simulink library "libMultiPacket"  (R2013b)
settings: Solver=ode45  StartTime=0.0  StopTime=10.0  RelTol=1e-3
undefined symbols (not defined in the file): macaddr
libraries: xpcutilitieslib x2, simulink x1, dspindex x1, libNetwork x1, xpcethernetlib x1, libSerialize x1
settings Model: Creator=djoshea  LastModifiedBy=djoshea

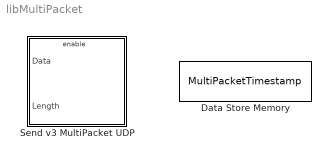
== system libMultiPacket ==
  Data Store Memory : DataStoreMemory  DataStoreName=MultiPacketTimestamp  ReadBeforeWriteMsg=warning  WriteAfterWriteMsg=warning  WriteAfterReadMsg=warning  OutDataTypeStr=double
  Send v3 MultiPacket UDP : Subsystem  mask{transmitId=1, sourceIP=[192 168 1 1], sourcePort=10000, destIP=[192 168 1 255], destPort=28000, DstMac=macaddr('ff:ff:ff:ff:ff:ff'), ID=1}
      mask prompts: transmitId "Transmit Block Id"; sourceIP "Source IP"; sourcePort "Source Port"; destIP "Dest IP"; destPort "Dest Port"; DstMac "Dest MAC"; ID "Ethernet Tx Id"
      mask TypeOptions sourceIP: Mask provides bytesPerPacket/sourceIP
      mask TypeOptions sourcePort: Mask provides bytesPerPacket/sourcePort
      mask TypeOptions destIP: Mask provides bytesPerPacket/destIP
      mask TypeOptions destPort: Mask provides bytesPerPacket/destPort
      mask TypeOptions DstMac: Mask provides bytesPerPacket/DstMac
      mask TypeOptions ID: Mask provides bytesPerPacket/ID

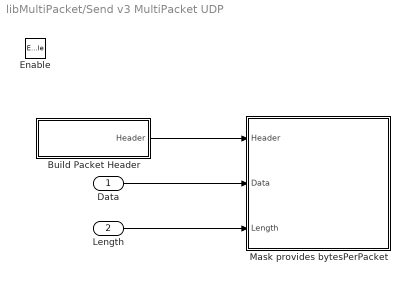
== system libMultiPacket/Send v3 MultiPacket UDP ==
  Data : Inport
  Length : Inport  Port=2  OutDataTypeStr=uint16
  Enable : EnablePort
  Build Packet Header : Subsystem
  Mask provides bytesPerPacket : Subsystem  mask{bytesPerPacket=1472-4-14, ID=1, sourceIP=sourceIP, sourcePort=10000, destIP=destIP, destPort=28000, DstMac=macaddr('ff:ff:ff:ff:ff:ff')}
      mask prompts: ID "Ethernet Tx Id"; sourceIP "Source IP"; sourcePort "Source Port"; destIP "Dest IP"; destPort "Dest Port"; DstMac "Dest MAC"
      mask TypeOptions ID: Packet Send Iterator/ID
      mask TypeOptions sourceIP: Packet Send Iterator/sourceIP
      mask TypeOptions sourcePort: Packet Send Iterator/sourcePort
      mask TypeOptions destIP: Packet Send Iterator/destIP
      mask TypeOptions destPort: Packet Send Iterator/destPort
      mask TypeOptions DstMac: Packet Send Iterator/DstMac
  wires:
  Build Packet Header/1(Header) -> Mask provides bytesPerPacket/1(Header)
  Length/1 -> Mask provides bytesPerPacket/3(Length)
  Data/1 -> Mask provides bytesPerPacket/2(Data)

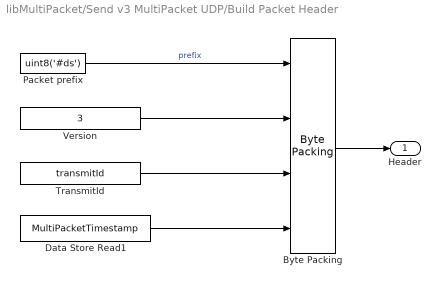
== system libMultiPacket/Send v3 MultiPacket UDP/Build Packet Header ==
  "Byte Packing " : xpcutilitieslib/Byte Packing   MaskPackedDataType=uint8  MaskUnpackedDataTypes={'uint8','uint16', 'uint8', 'double'}  MaskAlignment=1
  Data Store Read1 : DataStoreRead  DataStoreName=MultiPacketTimestamp
  Packet prefix : Constant  Value=uint8('#ds')  OutDataTypeStr=uint8
  TransmitId : Constant  Value=transmitId  OutDataTypeStr=uint8
  Version : Constant  Value=3  OutDataTypeStr=uint16
  Header : Outport
  wires:
  "Byte Packing "/1 -> Header/1
  Packet prefix/1 -> "Byte Packing "/1  "prefix"
  Version/1 -> "Byte Packing "/2
  Data Store Read1/1 -> "Byte Packing "/4
  TransmitId/1 -> "Byte Packing "/3

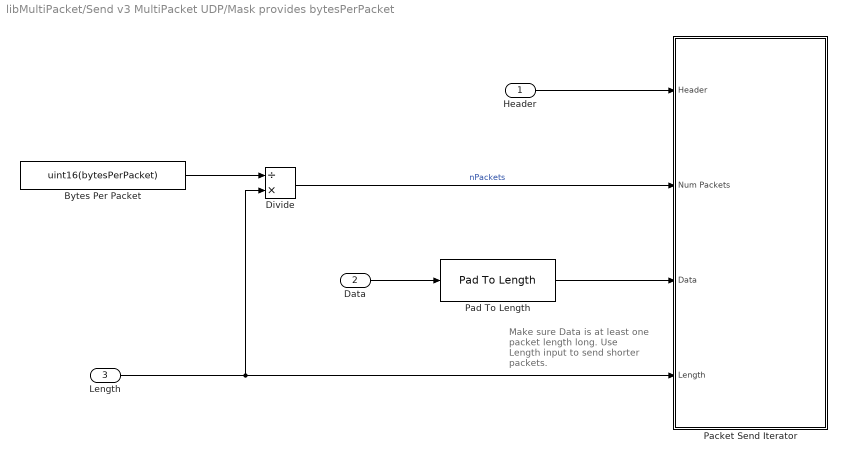
== system libMultiPacket/Send v3 MultiPacket UDP/Mask provides bytesPerPacket ==
  note: Make sure Data is at least one packet length long.
      | Use Length input to send shorter packets.
  Header : Inport
  Data : Inport  Port=2
  Length : Inport  Port=3  OutDataTypeStr=uint16
  Bytes Per Packet : Constant  Value=uint16(bytesPerPacket)  OutDataTypeStr=uint16
  Divide : Product  Inputs=/*  OutDataTypeStr=uint16  RndMeth=Ceiling
  Packet Send Iterator : Subsystem  TreatAsAtomicUnit=on  mask{bytesPerPacket=bytesPerPacket, ID=1, sourceIP=sourceIP, sourcePort=10000, destIP=destIP, destPort=28000, DstMac=macaddr('ff:ff:ff:ff:ff:ff')}
      mask prompts: bytesPerPacket "Bytes per Packet"; ID "Ethernet Tx Id"; sourceIP "Source IP"; sourcePort "Source Port"; destIP "Dest IP"; destPort "Dest Port"; DstMac "Dest MAC"
      mask TypeOptions ID: Send UDP/ID
      mask TypeOptions sourceIP: Send UDP/sourceIP
      mask TypeOptions sourcePort: Send UDP/sourcePort
      mask TypeOptions destIP: Send UDP/destIP
      mask TypeOptions destPort: Send UDP/destPort
      mask TypeOptions DstMac: Send UDP/DstMac
  Pad To Length : libSerialize/Pad To Length  bufferMinSize=bytesPerPacket
  wires:
  Header/1 -> Packet Send Iterator/1(Header)
  Pad To Length/1 -> Packet Send Iterator/3(Data)
  Divide/1 -> Packet Send Iterator/2(Num Packets)  "nPackets"
  Length/1 -> Packet Send Iterator/4(Length), Divide/2
  Bytes Per Packet/1 -> Divide/1
  Data/1 -> Pad To Length/1

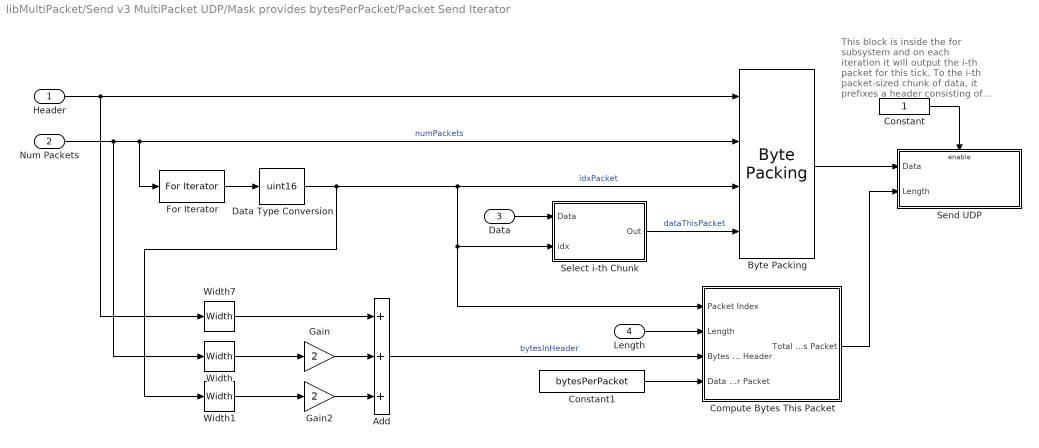
== system libMultiPacket/Send v3 MultiPacket UDP/Mask provides bytesPerPacket/Packet Send Iterator ==
  note: This block is inside the for subsystem and on each iteration
      | it will output the i-th packet for this tick. To the i-th packet-sized
      |  chunk of data, it prefixes a header consisting of a version, total
      |  packet count, and packet index.
  Header : Inport  OutDataTypeStr=uint8
  Num Packets : Inport  Port=2  OutDataTypeStr=uint16
  Data : Inport  Port=3  OutDataTypeStr=uint8
  Length : Inport  Port=4  OutDataTypeStr=uint16
  Add : Sum  Inputs=+++  OutDataTypeStr=uint16
  "Byte Packing " : xpcutilitieslib/Byte Packing   MaskPackedDataType=uint8  MaskUnpackedDataTypes={'uint8', 'uint16', 'uint16', 'uint8'}  MaskAlignment=1
  Compute Bytes This Packet : Subsystem
  Constant : Constant  OutDataTypeStr=Inherit: Inherit via back propagation
  Constant1 : Constant  Value=bytesPerPacket  OutDataTypeStr=uint16
  Data Type Conversion : DataTypeConversion  OutDataTypeStr=uint16
  For Iterator : ForIterator  IterationSource=external  IterationVariableDataType=int16
  Gain : Gain  Gain=2  OutDataTypeStr=uint16
  Gain2 : Gain  Gain=2  OutDataTypeStr=uint16
  Select i-th Chunk : Subsystem  mask{elementsPerChunk=bytesPerPacket}
      mask prompts: elementsPerChunk "Elements Per Chunk"
  Send UDP : Subsystem  mask{sourceIP=sourceIP, sourcePort=10000, destIP=destIP, destPort=28000, DstMac=macaddr('ff:ff:ff:ff:ff:ff'), ID=1}
      mask prompts: sourceIP "Source IP"; sourcePort "Source Port"; destIP "Dest IP"; destPort "Dest Port"; DstMac "Dest MAC"; ID "Ethernet Tx Id"
      mask TypeOptions sourceIP: sourceIP/Value
      mask TypeOptions sourcePort: sourcePort/Value
      mask TypeOptions destIP: destIP/Value
      mask TypeOptions destPort: destPort/Value
      mask TypeOptions DstMac: Build UDP Packet/DstMac
      mask TypeOptions ID: Ethernet Tx /ID
  Width : Width  DataType=uint16
  Width1 : Width  DataType=uint16
  Width7 : Width  DataType=uint16
  wires:
  Data Type Conversion/1 -> Select i-th Chunk/2(idx), Compute Bytes This Packet/1(Packet Index), "Byte Packing "/3, Width1/1  "idxPacket"
  Gain2/1 -> Add/3
  Header/1 -> "Byte Packing "/1, Width7/1
  Select i-th Chunk/1(Out) -> "Byte Packing "/4  "dataThisPacket"
  Constant/1 -> Send UDP/Enable
  Data/1 -> Select i-th Chunk/1(Data)
  For Iterator/1 -> Data Type Conversion/1
  Num Packets/1 -> For Iterator/1, "Byte Packing "/2, Width/1  "numPackets"
  "Byte Packing "/1 -> Send UDP/1(Data)
  Compute Bytes This Packet/1(Total Bytes This Packet) -> Send UDP/2(Length)
  Add/1 -> Compute Bytes This Packet/3(Bytes In Header)  "bytesInHeader"
  Length/1 -> Compute Bytes This Packet/2(Length)
  Width1/1 -> Gain2/1
  Gain/1 -> Add/2
  Width/1 -> Gain/1
  Width7/1 -> Add/1
  Constant1/1 -> Compute Bytes This Packet/4(Data Bytes Per Packet)

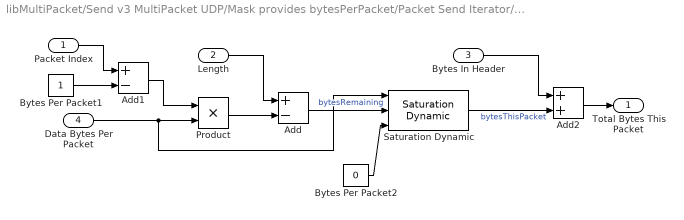
== system libMultiPacket/Send v3 MultiPacket UDP/Mask provides bytesPerPacket/Packet Send Iterator/Compute Bytes This Packet ==
  Packet Index : Inport  OutDataTypeStr=uint16
  Length : Inport  Port=2  OutDataTypeStr=uint16
  Bytes In Header : Inport  Port=3
  Data Bytes Per Packet : Inport  Port=4  OutDataTypeStr=uint16
  Add : Sum  Inputs=+-  OutDataTypeStr=Inherit: Same as first input
  Add1 : Sum  Inputs=+-  OutDataTypeStr=Inherit: Same as first input
  Add2 : Sum  OutDataTypeStr=Inherit: Same as first input
  Bytes Per Packet1 : Constant  OutDataTypeStr=uint16
  Bytes Per Packet2 : Constant  Value=0  OutDataTypeStr=uint16
  Product : Product  OutDataTypeStr=uint16  RndMeth=Zero
  Saturation Dynamic : simulink/Discontinuities/Saturation Dynamic  OutMin=[]  OutMax=[]  OutDataTypeStr=uint16  OutputDataTypeScalingMode=uint16  OutDataType=fixdt(1, 16)  OutScaling=2^-10  DoSatur=off
  Total Bytes This Packet : Outport  OutDataTypeStr=uint16
  wires:
  Data Bytes Per Packet/1 -> Product/2, Saturation Dynamic/1
  Add/1 -> Saturation Dynamic/2  "bytesRemaining"
  Product/1 -> Add/2
  Length/1 -> Add/1
  Add1/1 -> Product/1
  Bytes Per Packet1/1 -> Add1/2
  Saturation Dynamic/1 -> Add2/2  "bytesThisPacket"
  Packet Index/1 -> Add1/1
  Bytes In Header/1 -> Add2/1
  Add2/1 -> Total Bytes This Packet/1
  Bytes Per Packet2/1 -> Saturation Dynamic/3

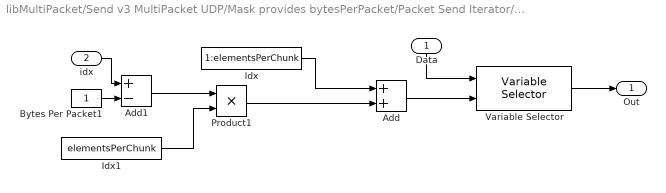
== system libMultiPacket/Send v3 MultiPacket UDP/Mask provides bytesPerPacket/Packet Send Iterator/Select i-th Chunk ==
  Data : Inport
  idx : Inport  Port=2
  Add : Sum  OutDataTypeStr=Inherit: Same as first input
  Add1 : Sum  Inputs=+-  OutDataTypeStr=Inherit: Same as first input
  Bytes Per Packet1 : Constant  OutDataTypeStr=uint16
  Idx : Constant  Value=1:elementsPerChunk
  Idx1 : Constant  Value=elementsPerChunk
  Product1 : Product  RndMeth=Zero  OutDataTypeStr=Inherit: Same as first input
  Variable Selector : dspindex/Variable Selector  NumInputs=1  rowsOrCols=Rows  IdxMode=Variable  Elements=[1 3]  ZerOneIdxMode=One-based  errmode=Generate Error  FillMode=off  FillValues=0
  Out : Outport
  wires:
  Idx1/1 -> Product1/2
  Idx/1 -> Add/1
  Product1/1 -> Add/2
  Add/1 -> Variable Selector/2
  Data/1 -> Variable Selector/1
  Variable Selector/1 -> Out/1
  Bytes Per Packet1/1 -> Add1/2
  idx/1 -> Add1/1
  Add1/1 -> Product1/1

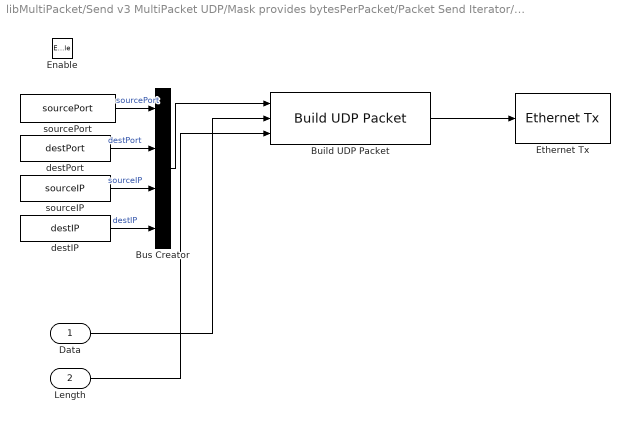
== system libMultiPacket/Send v3 MultiPacket UDP/Mask provides bytesPerPacket/Packet Send Iterator/Send UDP ==
  Data : Inport
  Length : Inport  Port=2
  Enable : EnablePort
  Build UDP Packet : libNetwork/Build UDP Packet  DstMac=macaddr('ff:ff:ff:ff:ff:ff')
  Bus Creator : BusCreator
  "Ethernet Tx " : xpcethernetlib/Ethernet Tx   ID=2  SampleTime=-1
  destIP : Constant  Value=destIP  VectorParams1D=off  OutDataTypeStr=uint8
  destPort : Constant  Value=destPort  VectorParams1D=off  OutDataTypeStr=uint16
  sourceIP : Constant  Value=sourceIP  VectorParams1D=off  OutDataTypeStr=uint8
  sourcePort : Constant  Value=sourcePort  VectorParams1D=off  OutDataTypeStr=uint16
  wires:
  Bus Creator/1 -> Build UDP Packet/1
  sourcePort/1 -> Bus Creator/1  "sourcePort"
  destPort/1 -> Bus Creator/2  "destPort"
  sourceIP/1 -> Bus Creator/3  "sourceIP"
  destIP/1 -> Bus Creator/4  "destIP"
  Length/1 -> Build UDP Packet/3
  Data/1 -> Build UDP Packet/2
  Build UDP Packet/1 -> "Ethernet Tx "/1
